simulink model "pannels"  (R2021a)
settings: Solver=VariableStepAuto  StartTime=0.0  StopTime=10.0  RelTol=1e-3
libraries: fl_lib x6, ee_lib x6
settings Model: Creator=yapudjus  LastModifiedBy=yapudjus

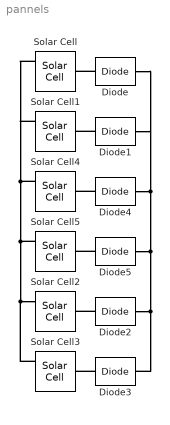
== system pannels ==
  Diode{,1..5} (6 alike) : fl_lib/Electrical/Electrical Elements/Diode  Vf=0.6 V  Ron=0.3 Ohm  Goff=1e-8 1/Ohm  i_specify=off  i_priority=None  i=0 A  i_nominal_specify=off  i_nominal_unit=A  i_nominal_value=1  v_specify=off  v_priority=None  v=0 V  v_nominal_specify=off  v_nominal_unit=V  v_nominal_value=1
  Solar Cell{,1..5} (6 alike) : ee_lib/Sources/Solar Cell  prm=1  Isc=9.72 A  Voc=21.6 V  Is=1e-6 A  Is2=0 A  Iph=7.34 A  Ir0=1000 W/m^2  ec=1.5  N2=2  Rs=0 Ohm  Rp=inf Ohm  N_series=1  TIPH1=0 1/K  EG=1.11 eV  TXIS1=3  TXIS2=3  TRS1=0  TRP1=0  Tmeas=25 degC  TFIXED=25 degC  thermal_mass=100 J/K  initial_temperature=25 degC
      settings: SourceProductBaseCode=PS
  connections:
  Diode/LConn1 -- Solar Cell/RConn1
  Diode1/LConn1 -- Solar Cell1/RConn1
  Solar Cell3/LConn2 -- Solar Cell1/LConn2 -- Solar Cell/LConn2 -- Solar Cell4/LConn2 -- Solar Cell5/LConn2 -- Solar Cell2/LConn2
  Diode3/LConn1 -- Solar Cell3/RConn1
  Diode2/LConn1 -- Solar Cell2/RConn1
  Diode4/RConn1 -- Diode5/RConn1 -- Diode3/RConn1 -- Diode2/RConn1 -- Diode1/RConn1 -- Diode/RConn1
  Diode5/LConn1 -- Solar Cell5/RConn1
  Diode4/LConn1 -- Solar Cell4/RConn1
